simulink model "Open_Loop_Closed_Loop_Second_order_system_respone_with_arduino"  (R2023a)
settings: Solver=FixedStepDiscrete  StartTime=0.0  StopTime=10  FixedStep=0.001  RelTol=1e-3  EnableMultiTasking=on
libraries: arduinolib x4
settings Model: ExtModeTrigDuration=2  Creator=Mohamed Ezzelrgal  LastModifiedBy=Mohamed Ezzelrgal
settings OptimizationCC: EnhancedBackFolding=on  PassReuseOutputArgsAs=Individual arguments  ZeroExternalMemoryAtStartup=off  ZeroInternalMemoryAtStartup=off  MaxStackSize=64  OptimizeBlockOrder=speed  DifferentSizesBufferReuse=on  OptimizationCustomize=off  EfficientTunableParamExpr=on
settings DebuggingCC: ParameterTunabilityLossMsg=error
settings HardwareCC: ProdBitPerInt=16  ProdBitPerPointer=16  ProdBitPerSizeT=16  ProdBitPerPtrDiffT=16  ProdLargestAtomicFloat=None  ProdWordSize=8  ProdHWDeviceType=Atmel->AVR
settings SFSimCC: MATLABDynamicMemAlloc=off
settings RTWCC: Description=Embedded Coder  SystemTargetFile=ert.tlc  HardwareBoard=Arduino Uno  TemplateMakefile=ert_default_tmf  Toolchain=Arduino AVR  BuildConfiguration=Faster Runs
settings CodeAppCC: ForceParamTrailComments=on  IgnoreCustomStorageClasses=off  OperatorAnnotations=on  SimulinkDataObjDesc=on  SFDataObjDesc=on  InsertBlockDesc=on
settings ERTTargetCC: SupportContinuousTime=on  SupportVariableSizeSignals=on  ExtModeTransport=3  ExtModeStaticAlloc=on  ExtModeAutomaticAllocSize=off  ExtModeStaticAllocSize=250  ExtModeMexFile=ext_xcp  ExtModeIntrfLevel=Level2 - Open

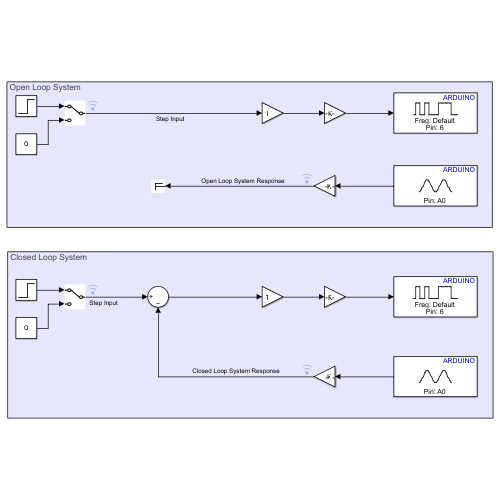
[thumbnail: Simulink's stored preview of the top-level diagram]
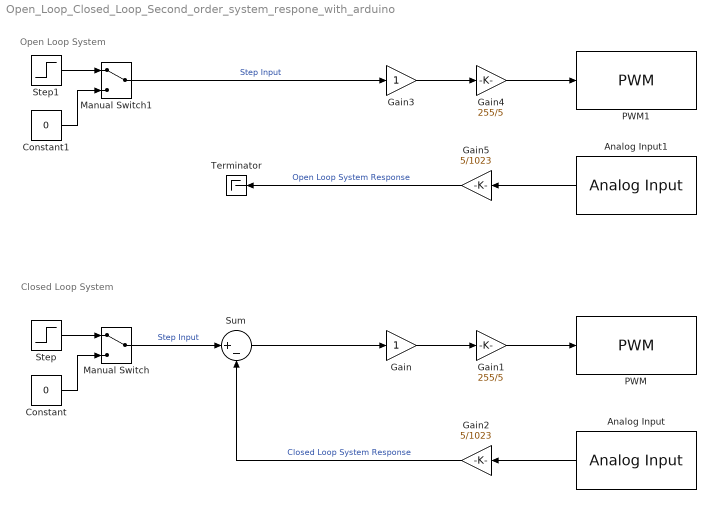
== system Open_Loop_Closed_Loop_Second_order_system_respone_with_arduino ==
  note: Closed Loop System
  note: Open Loop System
  Analog Input : arduinolib/Analog Input  pinNumber=0  ReadResultsOnly=off  ConversionTriggerSource=Software  ExternalTriggerType=uint32( 0 )  OutputDataType=uint16  EnableConversionCompleteNotify=off  EnableOuputStatus=off  SampleTime=-1  blockPlatform=arduino
  Analog Input1 : arduinolib/Analog Input  pinNumber=0  ReadResultsOnly=off  ConversionTriggerSource=Software  ExternalTriggerType=uint32( 0 )  OutputDataType=uint16  EnableConversionCompleteNotify=off  EnableOuputStatus=off  SampleTime=-1  blockPlatform=arduino
  Constant : Constant  Value=0
  Constant1 : Constant  Value=0
  Gain : Gain
  Gain1 : Gain  Gain=255/5
  Gain2 : Gain  Gain=5/1023
  Gain3 : Gain
  Gain4 : Gain  Gain=255/5
  Gain5 : Gain  Gain=5/1023
  Manual Switch : ManualSwitch
  Manual Switch1 : ManualSwitch
  PWM : arduinolib/PWM  pinNumber=6  frequencyType=Default  desiredFrequency=490.2  achievableFrequency=490.2
  PWM1 : arduinolib/PWM  pinNumber=6  frequencyType=Default  desiredFrequency=490.2  achievableFrequency=490.2
  Step : Step  SampleTime=0
  Step1 : Step  SampleTime=0
  Sum : Sum  Inputs=|+-
  Terminator : Terminator
  wires:
  Step/1 -> Manual Switch/1
  Gain/1 -> Gain1/1
  Gain1/1 -> PWM/1
  Constant/1 -> Manual Switch/2
  Analog Input/1 -> Gain2/1
  Gain2/1 -> Sum/2  "Closed Loop System Response"
  Manual Switch/1 -> Sum/1  "Step Input"
  Sum/1 -> Gain/1
  Manual Switch1/1 -> Gain3/1  "Step Input"
  Gain5/1 -> Terminator/1  "Open Loop System Response"
  Analog Input1/1 -> Gain5/1
  Constant1/1 -> Manual Switch1/2
  Gain4/1 -> PWM1/1
  Gain3/1 -> Gain4/1
  Step1/1 -> Manual Switch1/1
